simulink model "DDICBF_MO"  (R2022a)
settings: Solver=VariableStepAuto  StartTime=0.0  StopTime=50  FixedStep=0.01  RelTol=1e-3
values from neighbouring files (symbols this model uses):
  obs = [qO1,qO2]    [extract_MO.m]
  q1g = 1.9    [extract_MO.m]
  q2g = -0.8    [extract_MO.m]
  r = 0.5    [extract_MO.m]
  threshold_skip = 0.3    [extract_MO.m]
libraries: slctrlblks x1
settings Model: Creator=mirkomizzoni  LastModifiedBy=dennis

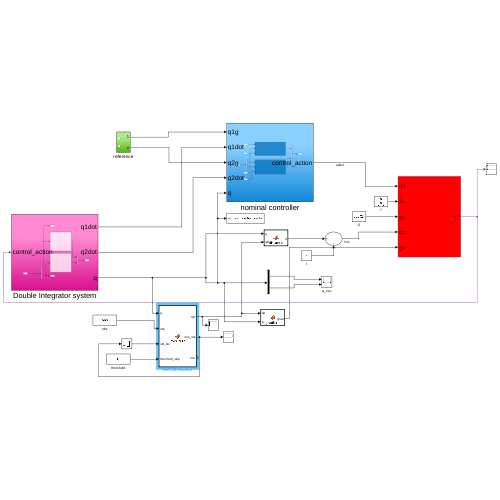
[thumbnail: Simulink's stored preview of the top-level diagram]
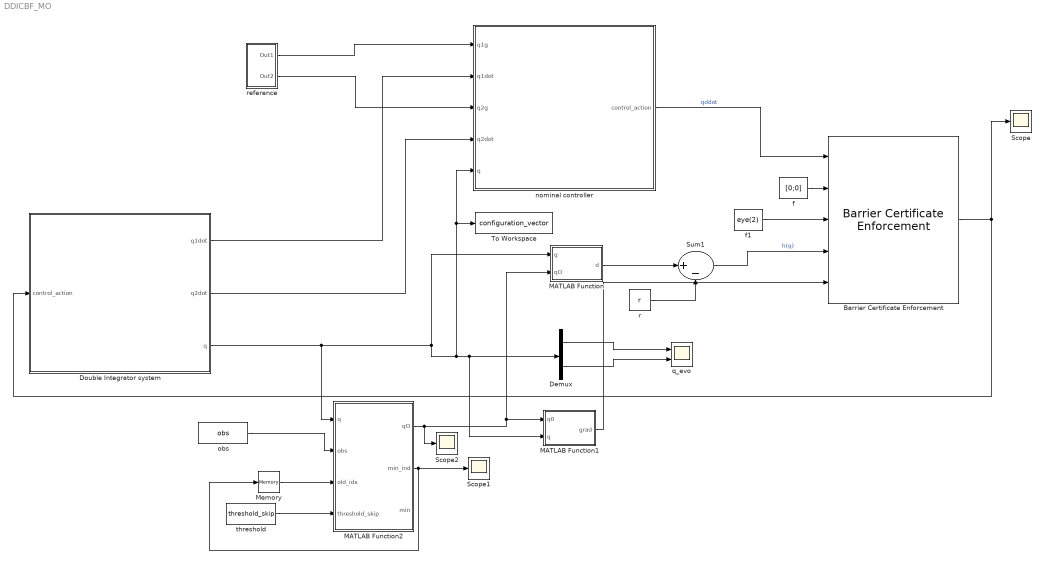
== system DDICBF_MO ==
  Barrier Certificate Enforcement : slctrlblks/Barrier Certificate Enforcement  nx=2  nu=2  nc=1  gamma=alpha  beta=1  external_umax=off  external_umin=off  Ts=0.1  maxiter=200  tol=1e-06  output_exitflag=off
      settings: SourceProductBaseCode=SD
  Demux : Demux  Outputs=2
  Double Integrator system : Subsystem
  MATLAB Function : MATLAB Function  TreatAsAtomicUnit=on
  MATLAB Function1 : MATLAB Function  TreatAsAtomicUnit=on
  MATLAB Function2 : MATLAB Function  TreatAsAtomicUnit=on
  Memory : Memory  InitialCondition=1
  Scope : Scope
  Scope1 : Scope
  Scope2 : Scope
  Sum1 : Sum  Inputs=|+-
  To Workspace : ToWorkspace  VariableName=configuration_vector  SaveFormat=Timeseries  SampleTime=-1
  f : Constant  Value=[0;0]  VectorParams1D=off
  f1 : Constant  Value=eye(2)  VectorParams1D=off
  nominal controller : Subsystem
  obs : Constant  Value=obs  VectorParams1D=off
  q_evo : Scope  NumInputPorts=2
  r : Constant  Value=r
  reference : Subsystem
  threshold : Constant  Value=threshold_skip  VectorParams1D=off
  wires:
  Demux/1 -> q_evo/1
  reference/2(Out2) -> nominal controller/3(q2g)
  reference/1(Out1) -> nominal controller/1(q1g)
  Barrier Certificate Enforcement/1 -> Double Integrator system/1(control_action), Scope/1
  MATLAB Function1/1(grad) -> Barrier Certificate Enforcement/5
  Demux/2 -> q_evo/2
  Sum1/1 -> Barrier Certificate Enforcement/4  "h(q)"
  nominal controller/1(control_action) -> Barrier Certificate Enforcement/1  "qddot"
  f1/1 -> Barrier Certificate Enforcement/3
  r/1 -> Sum1/2
  MATLAB Function/1(d) -> Sum1/1
  Double Integrator system/3(q) -> MATLAB Function1/2(q), Demux/1, To Workspace/1, nominal controller/5(q), MATLAB Function/1(q), MATLAB Function2/1(q)
  Double Integrator system/2(q2dot) -> nominal controller/4(q2dot)
  f/1 -> Barrier Certificate Enforcement/2
  Double Integrator system/1(q1dot) -> nominal controller/2(q1dot)
  obs/1 -> MATLAB Function2/2(obs)
  MATLAB Function2/1(qO) -> Scope2/1, MATLAB Function/2(qO), MATLAB Function1/1(q0)
  Memory/1 -> MATLAB Function2/3(old_idx)
  MATLAB Function2/2(min_ind) -> Scope1/1, Memory/1
  threshold/1 -> MATLAB Function2/4(threshold_skip)

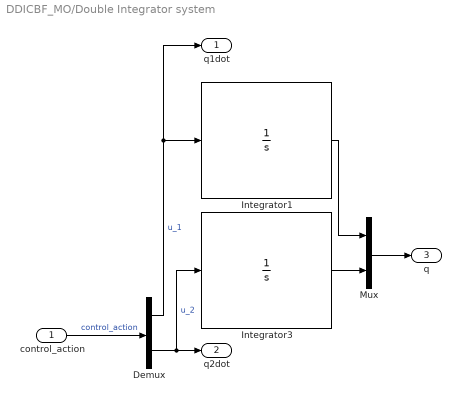
== system DDICBF_MO/Double Integrator system ==
  control_action : Inport
  Demux : Demux  Outputs=2
  Integrator1 : Integrator
  Integrator3 : Integrator
  Mux : Mux  Inputs=2
  q1dot : Outport
  q2dot : Outport  Port=2
  q : Outport  Port=3
  wires:
  Demux/1 -> q1dot/1, Integrator1/1  "u_1"
  Demux/2 -> q2dot/1, Integrator3/1  "u_2"
  Integrator1/1 -> Mux/1
  Integrator3/1 -> Mux/2
  control_action/1 -> Demux/1  "control_action"
  Mux/1 -> q/1

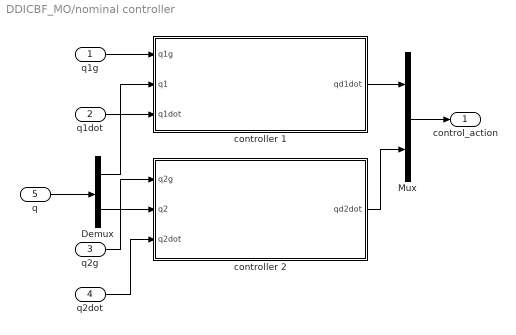
== system DDICBF_MO/nominal controller ==
  q1g : Inport
  q1dot : Inport  Port=2
  q2g : Inport  Port=3
  q2dot : Inport  Port=4
  q : Inport  Port=5
  Demux : Demux  Outputs=2
  Mux : Mux  Inputs=2
  controller 1 : Subsystem
  controller 2 : Subsystem
  control_action : Outport
  wires:
  controller 2/1(qd2dot) -> Mux/2
  controller 1/1(qd1dot) -> Mux/1
  q1g/1 -> controller 1/1(q1g)
  q2g/1 -> controller 2/1(q2g)
  Demux/2 -> controller 2/2(q2)
  Mux/1 -> control_action/1
  q2dot/1 -> controller 2/3(q2dot)
  Demux/1 -> controller 1/2(q1)
  q1dot/1 -> controller 1/3(q1dot)
  q/1 -> Demux/1

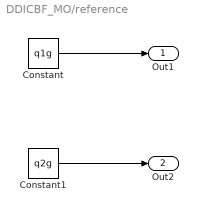
== system DDICBF_MO/reference ==
  Constant : Constant  Value=q1g
  Constant1 : Constant  Value=q2g
  Out1 : Outport
  Out2 : Outport  Port=2
  wires:
  Constant1/1 -> Out2/1
  Constant/1 -> Out1/1

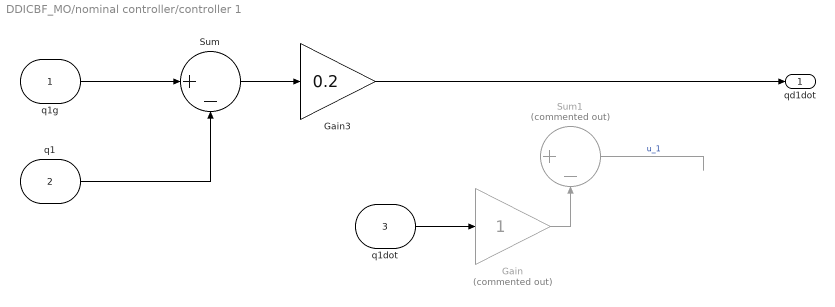
== system DDICBF_MO/nominal controller/controller 1 ==
  q1g : Inport
  q1 : Inport  Port=2
  q1dot : Inport  Port=3
  Gain : Gain  Commented=on
  Gain3 : Gain  Gain=0.2
  Sum : Sum  Inputs=|+-
  Sum1 : Sum  Commented=on  Inputs=|+-
  qd1dot : Outport
  wires:
  Sum1/1 -> ?  "u_1"
  q1/1 -> Sum/2
  Gain3/1 -> qd1dot/1
  Gain/1 -> Sum1/2
  Sum/1 -> Gain3/1
  q1g/1 -> Sum/1
  q1dot/1 -> Gain/1

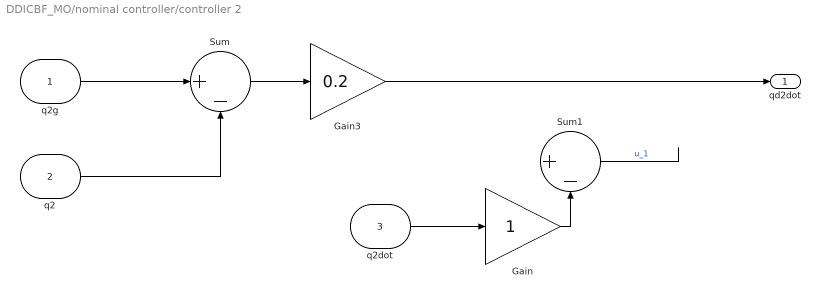
== system DDICBF_MO/nominal controller/controller 2 ==
  q2g : Inport
  q2 : Inport  Port=2
  q2dot : Inport  Port=3
  Gain : Gain
  Gain3 : Gain  Gain=0.2
  Sum : Sum  Inputs=|+-
  Sum1 : Sum  Inputs=|+-
  qd2dot : Outport
  wires:
  Sum1/1 -> ?  "u_1"
  Gain3/1 -> qd2dot/1
  Gain/1 -> Sum1/2
  Sum/1 -> Gain3/1
  q2g/1 -> Sum/1
  q2/1 -> Sum/2
  q2dot/1 -> Gain/1

== matlab function DDICBF_MO/MATLAB Function1 ==
  data: q0 input; grad output; q input
function grad = gradient(q0,q)
   grad = (q-q0)'/norm(q-q0);
end

== matlab function DDICBF_MO/MATLAB Function ==
  data: q input; qO input; d output
function d = distance(q,qO)
    d = norm(q-qO);
end

== matlab function DDICBF_MO/MATLAB Function2 ==
  data: q input; obs input; qO output; min_ind output; min output; old_idx input; threshold_skip input
function [qO,min_ind,min] = min_dist(q, obs, old_idx, threshold_skip)
[~,n] = size(obs);
min = norm(q-obs(:,1));
min_ind = 1;
for i=2:n
    t = norm(q-obs(:,i));
    if t<min
        min_ind = i;
        min = t;
    end
end

old_dist = norm(q-obs(:,old_idx));
if abs(old_dist-min) < threshold_skip
    qO = obs(:,old_idx);
    min_ind = old_idx;
    min = old_dist;
else
    qO = obs(:,min_ind);
end
